simulink subsystem "API020_PacketHandler"  (R2022b)
settings: Solver=VariableStepAuto  StartTime=0.0  StopTime=10.0  RelTol=1e-3
model mask{API020Period=WinMsgs.API020Period}
  mask prompts: API020Period "Packet Period"
settings Model: Creator=BEATOA  LastModifiedBy=BEATOA

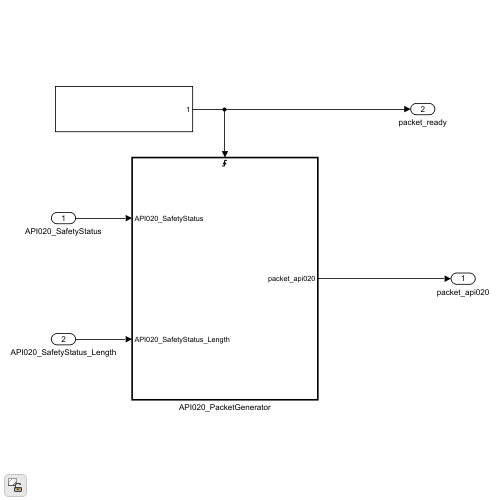
[thumbnail: Simulink's stored preview of the top-level diagram]
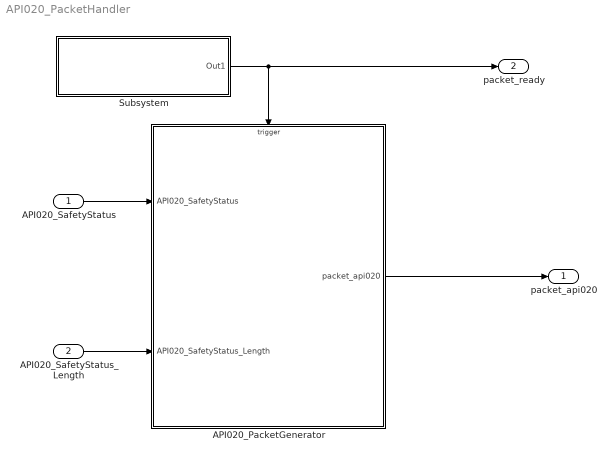
== system API020_PacketHandler ==
  API020_SafetyStatus : Inport
  API020_SafetyStatus_Length : Inport  Port=2
  API020_PacketGenerator : Subsystem
  Subsystem : Subsystem
  packet_api020 : Outport
  packet_ready : Outport  Port=2
  wires:
  API020_SafetyStatus_Length/1 -> API020_PacketGenerator/2(API020_SafetyStatus_Length)
  Subsystem/1(Out1) -> API020_PacketGenerator/Trigger, packet_ready/1
  API020_PacketGenerator/1(packet_api020) -> packet_api020/1
  API020_SafetyStatus/1 -> API020_PacketGenerator/1(API020_SafetyStatus)

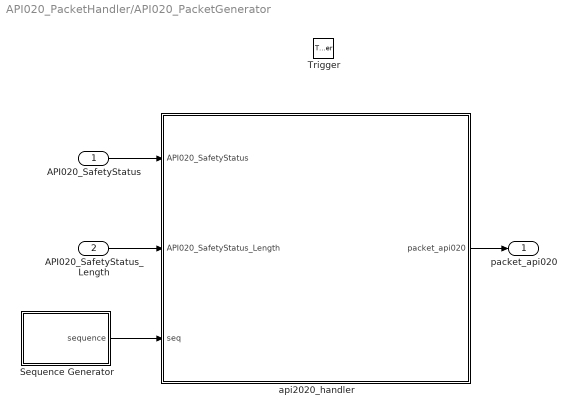
== system API020_PacketHandler/API020_PacketGenerator ==
  API020_SafetyStatus : Inport
  API020_SafetyStatus_Length : Inport  Port=2
  Trigger : TriggerPort  VariantControl=(inherit)  PortDimensions=1
  Sequence Generator : Subsystem
  api2020_handler : MATLAB Function  TreatAsAtomicUnit=on
  packet_api020 : Outport
  wires:
  Sequence Generator/1(sequence) -> api2020_handler/3(seq)
  API020_SafetyStatus_Length/1 -> api2020_handler/2(API020_SafetyStatus_Length)
  API020_SafetyStatus/1 -> api2020_handler/1(API020_SafetyStatus)
  api2020_handler/1(packet_api020) -> packet_api020/1

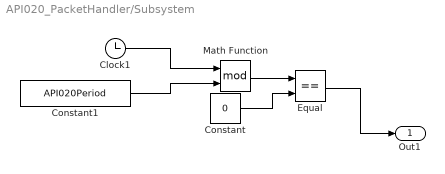
== system API020_PacketHandler/Subsystem ==
  Clock1 : Clock
  Constant : Constant  Value=0
  Constant1 : Constant  Value=API020Period
  Equal : RelationalOperator  Operator===  OutDataTypeStr=boolean  RndMeth=Simplest  InputSameDT=off
  Math Function : Math  Operator=mod
  Out1 : Outport
  wires:
  Constant1/1 -> Math Function/2
  Equal/1 -> Out1/1
  Math Function/1 -> Equal/1
  Constant/1 -> Equal/2
  Clock1/1 -> Math Function/1

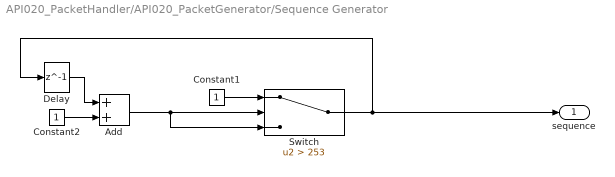
== system API020_PacketHandler/API020_PacketGenerator/Sequence Generator ==
  Add : Sum
  Constant1 : Constant
  Constant2 : Constant
  Delay : Delay  DelayLength=1  InitialCondition=1
  Switch : Switch  Criteria=u2 > Threshold  Threshold=253  SaturateOnIntegerOverflow=off  InputSameDT=off
  sequence : Outport
  wires:
  Add/1 -> Switch/2, Switch/3
  Constant1/1 -> Switch/1
  Delay/1 -> Add/1
  Constant2/1 -> Add/2
  Switch/1 -> Delay/1, sequence/1

== matlab function API020_PacketHandler/API020_PacketGenerator/api2020_handler ==
  data: API020_SafetyStatus input; API020_SafetyStatus_Length input; packet_api020 output; seq input
function packet_api020 = api2020(API020_SafetyStatus, API020_SafetyStatus_Length, seq)
    %% API020 Sequence
    packet_flags = flag_decoder(API020_SafetyStatus, API020_SafetyStatus_Length);  % would be good to create a decoding function from value to flags

    crc_dummy = 0; % Crc check on win packet not implemented
    
    % HEADER
    destination = 0;
    node_id = 1;
    destination_source = destination + node_id * (2^4);
    sdu_length = 7;
    sap = 4;
    api_id = 20;
    op_code = 2;
    cmd_fb = 1;
    frag = 0;
    mmp = 0;
    opcode_compl = op_code + cmd_fb * (2^5) + frag * (2^6) + mmp * (2^7);
    header_api020 = uint8([destination_source sap sdu_length api_id opcode_compl]);

    packet_api020 = zeros(100,1,'uint8');      
    temp = uint8([seq packet_flags ]);
    crc = CRCGen(temp);
    tmp = uint8([header_api020 temp crc crc_dummy]);
    packet_api020(1:length(tmp)) = tmp(:)';
end



function crc = CRCGen(data)
CRC8_TABLE =	['00'; '31'; '62'; '53'; 'C4'; 'F5'; 'A6'; '97'; ...
        'B9'; '88'; 'DB'; 'EA'; '7D'; '4C'; '1F'; '2E'; ...
        '43'; '72'; '21'; '10'; '87'; 'B6'; 'E5'; 'D4'; ...
        'FA'; 'CB'; '98'; 'A9'; '3E'; '0F'; '5C'; '6D'; ...
        '86'; 'B7'; 'E4'; 'D5'; '42'; '73'; '20'; '11'; ... 
        '3F'; '0E'; '5D'; '6C'; 'FB'; 'CA'; '99'; 'A8'; ...
        'C5'; 'F4'; 'A7'; '96'; '01'; '30'; '63'; '52'; ...
        '7C'; '4D'; '1E'; '2F'; 'B8'; '89'; 'DA'; 'EB'; ...
        '3D'; '0C'; '5F'; '6E'; 'F9'; 'C8'; '9B'; 'AA'; ...
        '84'; 'B5'; 'E6'; 'D7'; '40'; '71'; '22'; '13'; ...
        '7E'; '4F'; '1C'; '2D'; 'BA'; '8B'; 'D8'; 'E9'; ...
        'C7'; 'F6'; 'A5'; '94'; '03'; '32'; '61'; '50'; ...
        'BB'; '8A'; 'D9'; 'E8'; '7F'; '4E'; '1D'; '2C'; ...
        '02'; '33'; '60'; '51'; 'C6'; 'F7'; 'A4'; '95'; ...
        'F8'; 'C9'; '9A'; 'AB'; '3C'; '0D'; '5E'; '6F'; ...
        '41'; '70'; '23'; '12'; '85'; 'B4'; 'E7'; 'D6'; ...
        '7A'; '4B'; '18'; '29'; 'BE'; '8F'; 'DC'; 'ED'; ...
        'C3'; 'F2'; 'A1'; '90'; '07'; '36'; '65'; '54'; ...
        '39'; '08'; '5B'; '6A'; 'FD'; 'CC'; '9F'; 'AE'; ...
        '80'; 'B1'; 'E2'; 'D3'; '44'; '75'; '26'; '17'; ...
        'FC'; 'CD'; '9E'; 'AF'; '38'; '09'; '5A'; '6B'; ...
        '45'; '74'; '27'; '16'; '81'; 'B0'; 'E3'; 'D2'; ...
        'BF'; '8E'; 'DD'; 'EC'; '7B'; '4A'; '19'; '28'; ...
        '06'; '37'; '64'; '55'; 'C2'; 'F3'; 'A0'; '91'; ...
        '47'; '76'; '25'; '14'; '83'; 'B2'; 'E1'; 'D0'; ...
        'FE'; 'CF'; '9C'; 'AD'; '3A'; '0B'; '58'; '69'; ...
        '04'; '35'; '66'; '57'; 'C0'; 'F1'; 'A2'; '93'; ...
        'BD'; '8C'; 'DF'; 'EE'; '79'; '48'; '1B'; '2A'; ...
        'C1'; 'F0'; 'A3'; '92'; '05'; '34'; '67'; '56'; ...
        '78'; '49'; '1A'; '2B'; 'BC'; '8D'; 'DE'; 'EF'; ...
        '82'; 'B3'; 'E0'; 'D1'; '46'; '77'; '24'; '15'; ...
        '3B'; '0A'; '59'; '68'; 'FF'; 'CE'; '9D'; 'AC'];

    crc = uint8(255);
    for i = 1:length(data)
        arg = bitxor(crc,uint8(data(i)))+1;
        crc = uint8(hex2dec(CRC8_TABLE(arg,:)));
    end
end


function flags = flag_decoder(val, API020_SafetyStatus_Length)
    temp = zeros(1,API020_SafetyStatus_Length);
    for i = 1:API020_SafetyStatus_Length
        temp(i) = mod(val,2);
        val = bitshift(val,-1);
    end

    flags = temp;
end
